simulink model "ifoc_floueOBS"  (R2013a)
settings: Solver=ode45  StartTime=0.0  StopTime=tf  RelTol=1e-3
values from neighbouring files (symbols this model uses):
  A1 = A-(L*C)    [script_param.m]
  B = [(-P*0.85)/J;0]    [script_param.m]
  Cr = 0    [script_param.m]
  fr = 0.001    [script_param.m]
  FS = 50    [script_param.m]
  J = 0.2    [script_param.m]
  Lr = 0.1568    [script_param.m]
  Ls = 0.1568    [script_param.m]
  M = 0.15    [script_param.m]
  mm = L    [script_param.m]
  P = 2    [script_param.m]
  Rr = 1.8    [script_param.m]
  Rs = 1.2    [script_param.m]
  tcr = 3    [script_param.m]
  US = 230    [script_param.m]
libraries: fuzblock x3, simulink x1
settings Model: Creator=admin  LastModifiedBy=cyber
settings SolverCC: ZeroCrossControl=DisableAll
settings DebuggingCC: FrameProcessingCompatibilityMsg=error
settings GRTTargetCC: CodeReplacementLibrary=C89/C90 (ANSI)

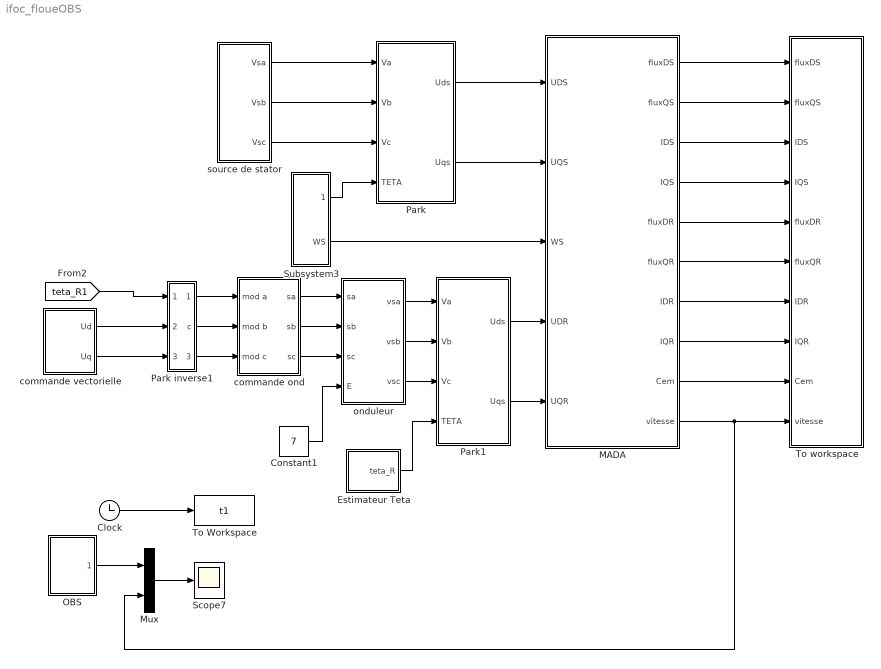
== system ifoc_floueOBS ==
  Clock : Clock
  Constant1 : Constant  Value=7
  Estimateur Teta : Subsystem
  MADA : Subsystem  mask{Rr=Rr, Lr=Lr, Rs=Rs, Ls=Ls, M=M, fr=fr, J=J, P=P, Cr=Cr, t1=tcr}
      mask prompts: t1 "tcr"
  Mux : Mux  Inputs=2
  OBS : Subsystem
  Park : Subsystem
  Park inverse1 : Subsystem
  Park1 : Subsystem
  Scope7 : Scope
      settings: TimeRange=0.0007659594403648384  MaxDataPoints=5000  SaveToWorkspace=off  YMin=153.447  YMax=153.448  SampleTime=-1
  Subsystem3 : Subsystem
  To Workspace : ToWorkspace  VariableName=t1  SaveFormat=Structure  SampleTime=-1
  To workspace : Subsystem
  commande ond : Subsystem
  commande vectorielle : Subsystem
  onduleur : Subsystem
  source de stator : Subsystem
  wires:
  Clock/1 -> To Workspace/1
  commande ond/1(sa) -> onduleur/1(sa)
  commande ond/2(sb) -> onduleur/2(sb)
  commande ond/3(sc) -> onduleur/3(sc)
  Constant1/1 -> onduleur/4(E)
  Park/1(Uds) -> MADA/1(UDS)
  Park/2(Uqs) -> MADA/2(UQS)
  source de stator/1(Vsa) -> Park/1("Va ")
  source de stator/2(Vsb) -> Park/2(Vb)
  source de stator/3(Vsc) -> Park/3(Vc)
  onduleur/1(vsa) -> Park1/1("Va ")
  onduleur/2(vsb) -> Park1/2(Vb)
  onduleur/3(vsc) -> Park1/3(Vc)
  Subsystem3/1(teta_S) -> Park/4(TETA)
  Estimateur Teta/1(teta_R) -> Park1/4(TETA)
  Subsystem3/2(WS) -> MADA/3(WS)
  Park1/1(Uds) -> MADA/4(UDR)
  Park1/2(Uqs) -> MADA/5(UQR)
  Park inverse1/1(a) -> commande ond/1(mod a)
  Park inverse1/2(c) -> commande ond/2(mod b)
  Park inverse1/3(b) -> commande ond/3(mod c)
  commande vectorielle/1(Ud) -> Park inverse1/2(d)
  commande vectorielle/2(Uq) -> Park inverse1/3(q)
  [teta_R1] -> Park inverse1/1(Teta)
  MADA/9(Cem) -> To workspace/9(Cem)
  MADA/8(IQR) -> To workspace/8(IQR)
  MADA/7(IDR) -> To workspace/7(IDR)
  MADA/6(fluxQR) -> To workspace/6(fluxQR)
  MADA/5(fluxDR) -> To workspace/5(fluxDR)
  MADA/4(IQS) -> To workspace/4(IQS)
  MADA/3(IDS) -> To workspace/3(IDS)
  MADA/2(fluxQS) -> To workspace/2(fluxQS)
  MADA/1(fluxDS) -> To workspace/1(fluxDS)
  MADA/10(vitesse) -> Mux/2, To workspace/10(vitesse)
  OBS/1(vit OBS) -> Mux/1
  Mux/1 -> Scope7/1

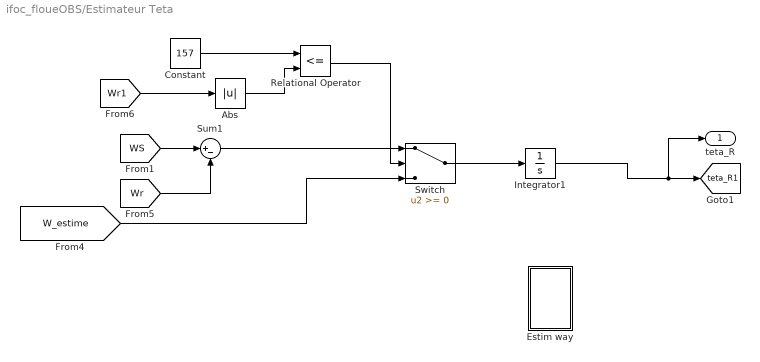
== system ifoc_floueOBS/Estimateur Teta ==
  Abs : Abs
  Constant : Constant  Value=157
  Estim way : Subsystem
  Integrator1 : Integrator
  Relational Operator : RelationalOperator  Operator=<=  OutDataTypeStr=boolean
  Sum1 : Sum  Inputs=|+-
  Switch : Switch
  teta_R : Outport
  tag scope: teta_R1=global
  wires:
  Integrator1/1 -> teta_R/1, [teta_R1]
  [WS] -> Sum1/1
  Constant/1 -> Relational Operator/1
  Relational Operator/1 -> Switch/2
  [W_estime] -> Switch/3
  [Wr1] -> Abs/1
  [Wr] -> Sum1/2
  Sum1/1 -> Switch/1
  Abs/1 -> Relational Operator/2
  Switch/1 -> Integrator1/1

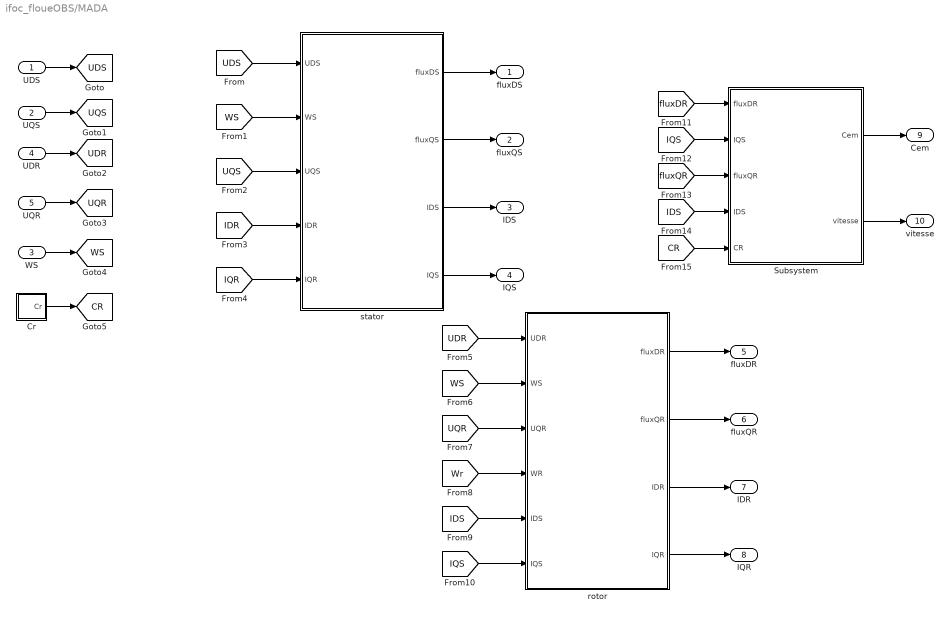
== system ifoc_floueOBS/MADA ==
  UDS : Inport
  UQS : Inport  Port=2
  WS : Inport  Port=3
  UDR : Inport  Port=4
  UQR : Inport  Port=5
  Cr : Subsystem
  Subsystem : Subsystem
  rotor : Subsystem
  stator : Subsystem
  fluxDS : Outport
  fluxQS : Outport  Port=2
  IDS : Outport  Port=3
  IQS : Outport  Port=4
  fluxDR : Outport  Port=5
  fluxQR : Outport  Port=6
  IDR : Outport  Port=7
  IQR : Outport  Port=8
  Cem : Outport  Port=9
  vitesse : Outport  Port=10
  tag scope: CR=global, UDR=global, UDS=global, UQR=global, UQS=global, WS=global
  wires:
  UDS/1 -> [UDS]
  UQS/1 -> [UQS]
  UDR/1 -> [UDR]
  WS/1 -> [WS]
  stator/1(fluxDS) -> fluxDS/1
  stator/2(fluxQS) -> fluxQS/1
  stator/3(IDS) -> IDS/1
  stator/4(IQS) -> IQS/1
  Subsystem/1(Cem) -> Cem/1
  Subsystem/2(vitesse) -> vitesse/1
  rotor/1(fluxDR) -> fluxDR/1
  rotor/2(fluxQR) -> fluxQR/1
  rotor/3(IDR) -> IDR/1
  rotor/4(IQR) -> IQR/1
  [UDS] -> stator/1(UDS)
  [WS] -> stator/2(WS)
  [UQS] -> stator/3(UQS)
  [IDR] -> stator/4(IDR)
  [IQR] -> stator/5(IQR)
  [UDR] -> rotor/1(UDR)
  [WS] -> rotor/2(WS)
  [UQR] -> rotor/3(UQR)
  [Wr] -> rotor/4(WR)
  [IDS] -> rotor/5(IDS)
  [IQS] -> rotor/6(IQS)
  [fluxDR] -> Subsystem/1(fluxDR)
  [IQS] -> Subsystem/2(IQS)
  [fluxQR] -> Subsystem/3(fluxQR)
  [IDS] -> Subsystem/4(IDS)
  [CR] -> Subsystem/5(CR)
  Cr/1(Cr) -> [CR]
  UQR/1 -> [UQR]

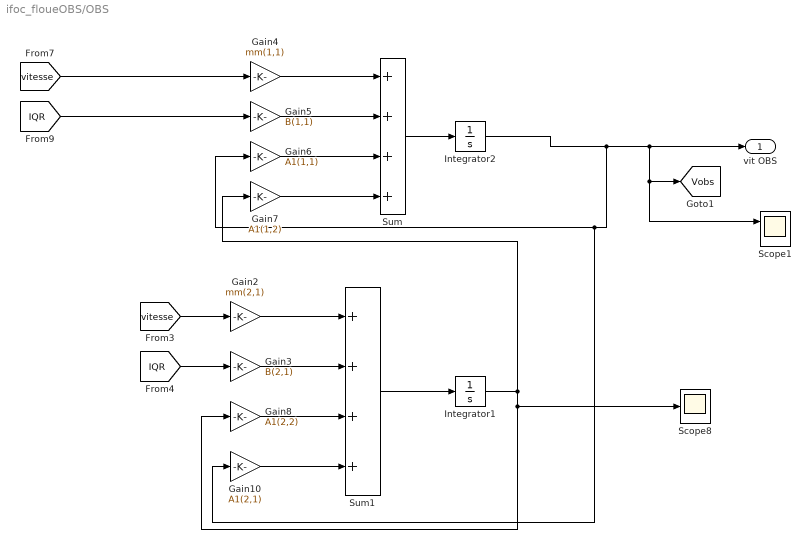
== system ifoc_floueOBS/OBS ==
  Gain10 : Gain  Gain=A1(2,1)
  Gain2 : Gain  Gain=mm(2,1)
  Gain3 : Gain  Gain=B(2,1)
  Gain4 : Gain  Gain=mm(1,1)
  Gain5 : Gain  Gain=B(1,1)
  Gain6 : Gain  Gain=A1(1,1)
  Gain7 : Gain  Gain=A1(1,2)
  Gain8 : Gain  Gain=A1(2,2)
  Integrator1 : Integrator
  Integrator2 : Integrator
  Scope1 : Scope  NumInputPorts=2
      settings: TimeRange=0.0007659594403648384  MaxDataPoints=5000  SaveToWorkspace=off  SaveName=ScopeData31  YMin=153.447~-5  YMax=153.448~5  SampleTime=-1
  Scope8 : Scope
      settings: TimeRange=0.0007659594403648384  MaxDataPoints=5000  SaveToWorkspace=off  SaveName=ScopeData43  YMin=156.9  YMax=157  SampleTime=-1
  Sum : Sum  Inputs=++++
  Sum1 : Sum  Inputs=++++
  vit OBS : Outport
  tag scope: Vobs=global
  wires:
  [vitesse] -> Gain4/1
  [IQR] -> Gain5/1
  Sum/1 -> Integrator2/1
  Integrator2/1 -> Gain10/1, Gain6/1, Scope1/1, [Vobs], vit OBS/1
  Gain7/1 -> Sum/4
  Gain6/1 -> Sum/3
  Gain5/1 -> Sum/2
  Gain4/1 -> Sum/1
  Sum1/1 -> Integrator1/1
  Integrator1/1 -> Gain7/1, Gain8/1, Scope8/1
  [IQR] -> Gain3/1
  Gain3/1 -> Sum1/2
  Gain8/1 -> Sum1/3
  Gain10/1 -> Sum1/4
  [vitesse] -> Gain2/1
  Gain2/1 -> Sum1/1

== system ifoc_floueOBS/Park ==
  "Va " : Inport
  Vb : Inport  Port=2
  Vc : Inport  Port=3
  TETA : Inport  Port=4
  Scope : Scope  NumInputPorts=2
      settings: TimeRange=0.02  LimitDataPoints=on  MaxDataPoints=5000  SaveToWorkspace=off  SaveName=ScopeData  YMin=-0.1~-9.311418685121105e+25  YMax=1~-7.437818033787908e+25  SampleTime=-1
  Transformation de Park : Subsystem
  Uds : Outport
  Uqs : Outport  Port=2
  wires:
  Transformation de Park/2(q) -> Uqs/1, Scope/2
  Transformation de Park/1(d) -> Uds/1, Scope/1
  "Va "/1 -> Transformation de Park/1(Va)
  Vb/1 -> Transformation de Park/2(Vb)
  Vc/1 -> Transformation de Park/3(Vc)
  TETA/1 -> Transformation de Park/4(TETA)

== system ifoc_floueOBS/Park inverse1 ==
  Teta : Inport
  d : Inport  Port=2
  q : Inport  Port=3
  Transformer alpha/betta : Subsystem
  Transformer dq : Subsystem
  a : Outport
  c : Outport  Port=2
  b : Outport  Port=3
  wires:
  q/1 -> Transformer alpha/betta/3(Iq)
  d/1 -> Transformer alpha/betta/2(Id)
  Teta/1 -> Transformer alpha/betta/1(Teta)
  Transformer dq/3(Ic) -> c/1
  Transformer dq/2(Ib) -> b/1
  Transformer dq/1(Ia) -> a/1
  Transformer alpha/betta/2(Xbeta) -> Transformer dq/2(Xbeta)
  Transformer alpha/betta/1(Xalpha) -> Transformer dq/1(Xalpha)

== system ifoc_floueOBS/Park1 ==
  "Va " : Inport
  Vb : Inport  Port=2
  Vc : Inport  Port=3
  TETA : Inport  Port=4
  Scope : Scope  NumInputPorts=2
      settings: TimeRange=0.02  LimitDataPoints=on  MaxDataPoints=5000  SaveToWorkspace=off  SaveName=ScopeData  YMin=-0.1~-9.311418685121105e+25  YMax=1~-7.437818033787908e+25  SampleTime=-1
  Transformation de Park : Subsystem
  Uds : Outport
  Uqs : Outport  Port=2
  wires:
  TETA/1 -> Transformation de Park/4(TETA)
  Vc/1 -> Transformation de Park/3(Vc)
  Vb/1 -> Transformation de Park/2(Vb)
  "Va "/1 -> Transformation de Park/1(Va)
  Transformation de Park/1(d) -> Scope/1, Uds/1
  Transformation de Park/2(q) -> Scope/2, Uqs/1

== system ifoc_floueOBS/Subsystem3 ==
  Constant2 : Constant  Value=2*pi*50
  Integrator2 : Integrator
  teta_S : Outport
  WS : Outport  Port=2
  tag scope: teta_S=global
  wires:
  Integrator2/1 -> [teta_S], teta_S/1
  Constant2/1 -> Integrator2/1
  [Wr1] -> WS/1

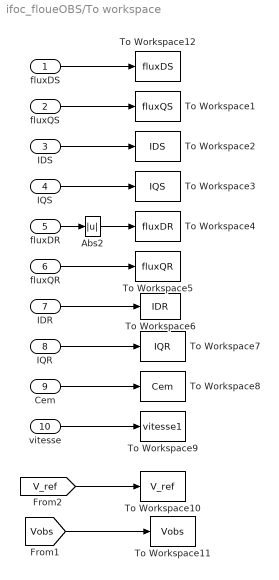
== system ifoc_floueOBS/To workspace ==
  fluxDS : Inport
  fluxQS : Inport  Port=2
  IDS : Inport  Port=3
  IQS : Inport  Port=4
  fluxDR : Inport  Port=5
  fluxQR : Inport  Port=6
  IDR : Inport  Port=7
  IQR : Inport  Port=8
  Cem : Inport  Port=9
  vitesse : Inport  Port=10
  Abs2 : Abs
  To Workspace1 : ToWorkspace  VariableName=fluxQS  SaveFormat=Structure  SampleTime=-1
  To Workspace10 : ToWorkspace  VariableName=V_ref  SaveFormat=Structure  SampleTime=-1
  To Workspace11 : ToWorkspace  VariableName=Vobs  SaveFormat=Structure  SampleTime=-1
  To Workspace12 : ToWorkspace  VariableName=fluxDS  SaveFormat=Structure  SampleTime=-1
  To Workspace2 : ToWorkspace  VariableName=IDS  SaveFormat=Structure  SampleTime=-1
  To Workspace3 : ToWorkspace  VariableName=IQS  SaveFormat=Structure  SampleTime=-1
  To Workspace4 : ToWorkspace  VariableName=fluxDR  SaveFormat=Structure  SampleTime=-1
  To Workspace5 : ToWorkspace  VariableName=fluxQR  SaveFormat=Structure  SampleTime=-1
  To Workspace6 : ToWorkspace  VariableName=IDR  SaveFormat=Structure  SampleTime=-1
  To Workspace7 : ToWorkspace  VariableName=IQR  SaveFormat=Structure  SampleTime=-1
  To Workspace8 : ToWorkspace  VariableName=Cem  SaveFormat=Structure  SampleTime=-1
  To Workspace9 : ToWorkspace  VariableName=vitesse1  SaveFormat=Structure  SampleTime=-1
  wires:
  fluxDS/1 -> To Workspace12/1
  fluxQS/1 -> To Workspace1/1
  IDS/1 -> To Workspace2/1
  IQS/1 -> To Workspace3/1
  fluxQR/1 -> To Workspace5/1
  IQR/1 -> To Workspace7/1
  Cem/1 -> To Workspace8/1
  vitesse/1 -> To Workspace9/1
  fluxDR/1 -> Abs2/1
  Abs2/1 -> To Workspace4/1
  [V_ref] -> To Workspace10/1
  IDR/1 -> To Workspace6/1
  [Vobs] -> To Workspace11/1

== system ifoc_floueOBS/commande ond ==
  mod a : Inport
  mod b : Inport  Port=2
  mod c : Inport  Port=3
  Data Type Conversion : DataTypeConversion  SaturateOnIntegerOverflow=on  RndMeth=Zero
  Data Type Conversion1 : DataTypeConversion  SaturateOnIntegerOverflow=on  RndMeth=Zero
  Data Type Conversion2 : DataTypeConversion  SaturateOnIntegerOverflow=on  RndMeth=Zero
  Relational Operator : RelationalOperator  OutDataTypeStr=boolean
  Relational Operator1 : RelationalOperator  OutDataTypeStr=boolean
  Relational Operator2 : RelationalOperator  OutDataTypeStr=boolean
  Repeating Sequence : simulink/Sources/Repeating Sequence  rep_seq_t="[0 1e-3/4 1e-3/2 3e-3/4  1e-3]"  rep_seq_y="[0 320 0 -320  0]"
  sa : Outport
  sb : Outport  Port=2
  sc : Outport  Port=3
  wires:
  Repeating Sequence/1 -> Relational Operator1/2, Relational Operator/2, Relational Operator2/2
  mod b/1 -> Relational Operator1/1
  mod c/1 -> Relational Operator2/1
  Relational Operator/1 -> Data Type Conversion/1
  Relational Operator1/1 -> Data Type Conversion1/1
  Relational Operator2/1 -> Data Type Conversion2/1
  Data Type Conversion/1 -> sa/1
  Data Type Conversion1/1 -> sb/1
  Data Type Conversion2/1 -> sc/1
  mod a/1 -> Relational Operator/1

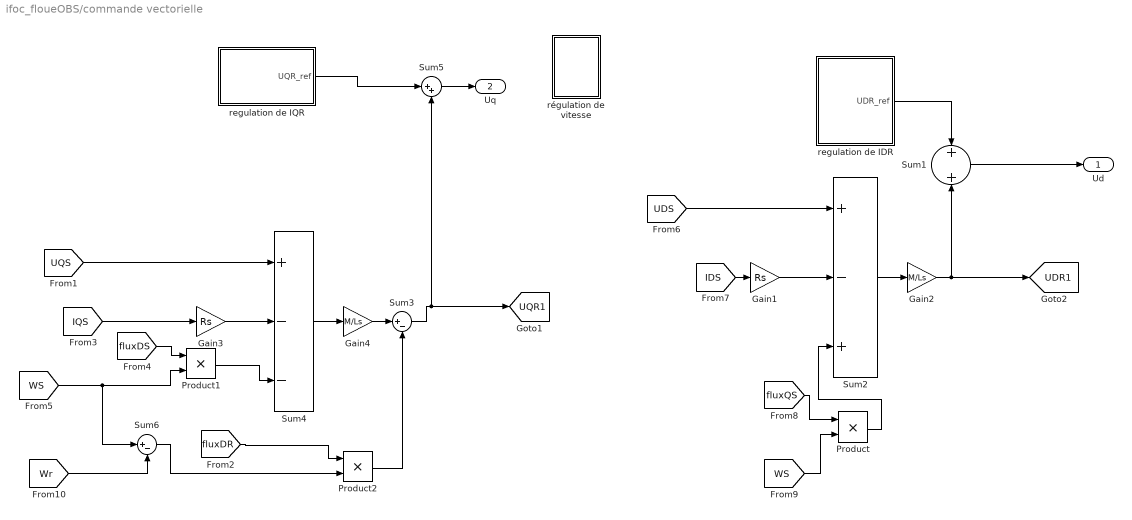
== system ifoc_floueOBS/commande vectorielle ==
  Gain1 : Gain  Gain=Rs
  Gain2 : Gain  Gain=M/Ls
  Gain3 : Gain  Gain=Rs
  Gain4 : Gain  Gain=M/Ls
  Product : Product
  Product1 : Product
  Product2 : Product
  Sum1 : Sum
  Sum2 : Sum  Inputs=+-+
  Sum3 : Sum  Inputs=|+-
  Sum4 : Sum  Inputs=+--
  Sum5 : Sum  Inputs=|++
  Sum6 : Sum  Inputs=|+-
  regulation de IDR : Subsystem
  regulation de IQR : Subsystem
  "régulation de vitesse " : Subsystem
  Ud : Outport
  Uq : Outport  Port=2
  tag scope: UDR1=global, UQR1=global
  wires:
  [fluxQS] -> Product/1
  [IDS] -> Gain1/1
  [UDS] -> Sum2/1
  Gain1/1 -> Sum2/2
  Product/1 -> Sum2/3
  Sum2/1 -> Gain2/1
  [WS] -> Product/2
  Gain2/1 -> Sum1/2, [UDR1]
  Sum1/1 -> Ud/1
  regulation de IDR/1(UDR_ref) -> Sum1/1
  Sum4/1 -> Gain4/1
  Product1/1 -> Sum4/3
  Gain3/1 -> Sum4/2
  [UQS] -> Sum4/1
  [IQS] -> Gain3/1
  [WS] -> Product1/2, Sum6/1
  [fluxDS] -> Product1/1
  Product2/1 -> Sum3/2
  [fluxDR] -> Product2/1
  Gain4/1 -> Sum3/1
  [Wr] -> Sum6/2
  Sum6/1 -> Product2/2
  regulation de IQR/1(UQR_ref) -> Sum5/1
  Sum3/1 -> [UQR1], Sum5/2
  Sum5/1 -> Uq/1

== system ifoc_floueOBS/onduleur ==
  sa : Inport
  sb : Inport  Port=2
  sc : Inport  Port=3
  E : Inport  Port=4
  Mux : Mux
  Va : Fcn  Expr=u(4)*((2/3)*u(1)+(-1/3)*u(2)+(-1/3)*u(3))
  Vb : Fcn  Expr=u(4)*((-1/3)*u(1)+(2/3)*u(2)-(1/3)*u(3))
  Vc : Fcn  Expr=u(4)*((-1/3)*u(1)-(1/3)*u(2)+(2/3)*u(3))
  vsa : Outport
  vsb : Outport  Port=2
  vsc : Outport  Port=3
  wires:
  sa/1 -> Mux/1
  sb/1 -> Mux/2
  sc/1 -> Mux/3
  Mux/1 -> Va/1, Vb/1, Vc/1
  Va/1 -> vsa/1
  Vb/1 -> vsb/1
  Vc/1 -> vsc/1
  E/1 -> Mux/4

== system ifoc_floueOBS/source de stator ==
  Sine Wave : Sin  Amplitude=US  Frequency=FS*2*pi  SampleTime=0
  Sine Wave1 : Sin  Amplitude=US  Frequency=FS*2*pi  Phase=-2*pi/3  SampleTime=0
  Sine Wave2 : Sin  Amplitude=US  Frequency=FS*2*pi  Phase=-4*pi/3  SampleTime=0
  Vsa : Outport
  Vsb : Outport  Port=2
  Vsc : Outport  Port=3
  wires:
  Sine Wave2/1 -> Vsc/1
  Sine Wave1/1 -> Vsb/1
  Sine Wave/1 -> Vsa/1

== system ifoc_floueOBS/Estimateur Teta/Estim way ==
  Constant1 : Constant  Value=0.85
  Gain : Gain  Gain=Rr
  Product : Product  Inputs=*/
  Sum : Sum  Inputs=+-
  tag scope: W_estime=global
  wires:
  [IQR] -> Gain/1
  [UQR] -> Sum/1
  Gain/1 -> Sum/2
  Sum/1 -> Product/1
  Product/1 -> [W_estime]
  Constant1/1 -> Product/2

== system ifoc_floueOBS/MADA/Cr ==
  Step : Step  Time=tcr  After=Cr  SampleTime=0
  Cr : Outport
  wires:
  Step/1 -> Cr/1

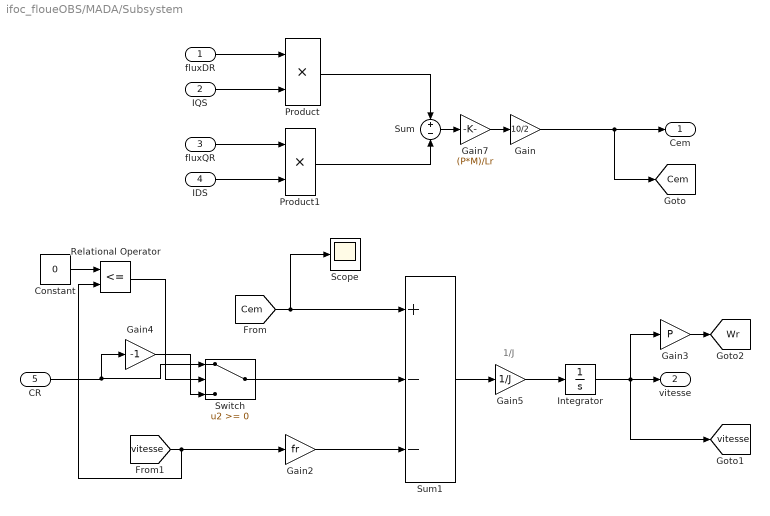
== system ifoc_floueOBS/MADA/Subsystem ==
  note: 1/J
  fluxDR : Inport
  IQS : Inport  Port=2
  fluxQR : Inport  Port=3
  IDS : Inport  Port=4
  CR : Inport  Port=5
  Constant : Constant  Value=0
  Gain : Gain  Gain=10/2
  Gain2 : Gain  Gain=fr
  Gain3 : Gain  Gain=P
  Gain4 : Gain  Gain=-1
  Gain5 : Gain  Gain=1/J
  Gain7 : Gain  Gain=(P*M)/Lr
  Integrator : Integrator
  Product : Product
  Product1 : Product
  Relational Operator : RelationalOperator  Operator=<=  OutDataTypeStr=boolean
  Scope : Scope
      settings: TimeRange=auto  MaxDataPoints=5000  SaveToWorkspace=off  SaveName=ScopeData4  YMin=-10  YMax=10  SampleTime=-1
  Sum : Sum  Inputs=+|-
  Sum1 : Sum  Inputs=+--
  Switch : Switch
  Cem : Outport
  vitesse : Outport  Port=2
  tag scope: Cem=global, Wr=global, vitesse=global
  wires:
  fluxDR/1 -> Product/1
  IQS/1 -> Product/2
  IDS/1 -> Product1/2
  fluxQR/1 -> Product1/1
  Sum/1 -> Gain7/1
  Gain/1 -> [Cem], Cem/1
  [vitesse] -> Relational Operator/2, Gain2/1
  Gain3/1 -> [Wr]
  Integrator/1 -> vitesse/1, Gain3/1, [vitesse]
  Constant/1 -> Relational Operator/1
  Relational Operator/1 -> Switch/2
  Gain4/1 -> Switch/3
  Sum1/1 -> Gain5/1
  Gain5/1 -> Integrator/1
  Gain2/1 -> Sum1/3
  Product1/1 -> Sum/2
  Product/1 -> Sum/1
  Gain7/1 -> Gain/1
  [Cem] -> Sum1/1, Scope/1
  CR/1 -> Switch/1, Gain4/1
  Switch/1 -> Sum1/2

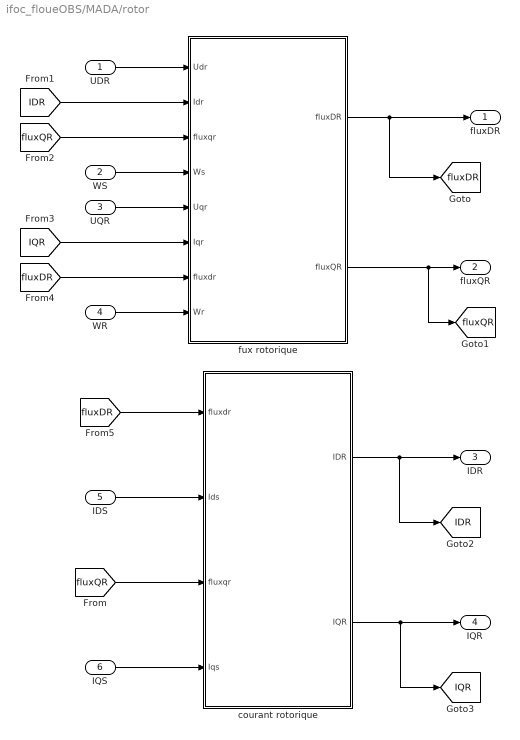
== system ifoc_floueOBS/MADA/rotor ==
  UDR : Inport
  WS : Inport  Port=2
  UQR : Inport  Port=3
  WR : Inport  Port=4
  IDS : Inport  Port=5
  IQS : Inport  Port=6
  courant rotorique : Subsystem
  fux rotorique : Subsystem
  fluxDR : Outport
  fluxQR : Outport  Port=2
  IDR : Outport  Port=3
  IQR : Outport  Port=4
  tag scope: IDR=global, IQR=global, fluxDR=global, fluxQR=global
  wires:
  courant rotorique/1(IDR) -> [IDR], IDR/1
  courant rotorique/2(IQR) -> [IQR], IQR/1
  UDR/1 -> fux rotorique/1(Udr)
  WS/1 -> fux rotorique/4(Ws)
  UQR/1 -> fux rotorique/5(Uqr)
  WR/1 -> fux rotorique/8(Wr)
  IDS/1 -> courant rotorique/2(Ids)
  IQS/1 -> courant rotorique/4(Iqs)
  [IDR] -> fux rotorique/2(Idr)
  [fluxQR] -> fux rotorique/3(fluxqr)
  [IQR] -> fux rotorique/6(Iqr)
  [fluxDR] -> fux rotorique/7(fluxdr)
  [fluxDR] -> courant rotorique/1(fluxdr)
  [fluxQR] -> courant rotorique/3(fluxqr)
  fux rotorique/2(fluxQR) -> [fluxQR], fluxQR/1
  fux rotorique/1(fluxDR) -> fluxDR/1, [fluxDR]

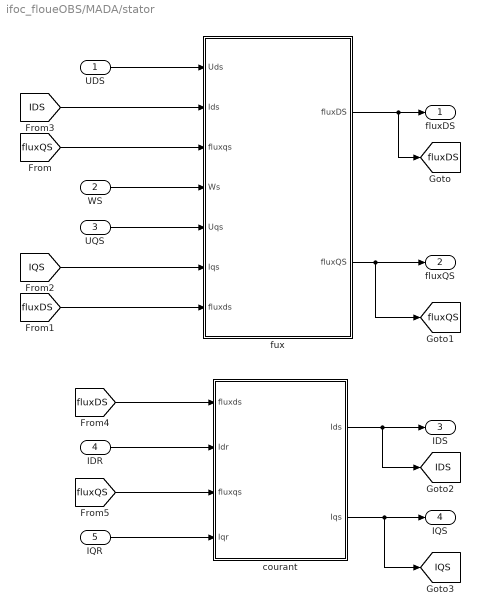
== system ifoc_floueOBS/MADA/stator ==
  UDS : Inport
  WS : Inport  Port=2
  UQS : Inport  Port=3
  IDR : Inport  Port=4
  IQR : Inport  Port=5
  "courant " : Subsystem
  fux : Subsystem
  fluxDS : Outport
  fluxQS : Outport  Port=2
  IDS : Outport  Port=3
  IQS : Outport  Port=4
  tag scope: IDS=global, IQS=global, fluxDS=global, fluxQS=global
  wires:
  fux/1(fluxDS) -> [fluxDS], fluxDS/1
  fux/2(fluxQS) -> [fluxQS], fluxQS/1
  "courant "/1(Ids) -> [IDS], IDS/1
  "courant "/2(Iqs) -> [IQS], IQS/1
  UDS/1 -> fux/1(Uds)
  WS/1 -> fux/4(Ws)
  UQS/1 -> fux/5(Uqs)
  IDR/1 -> "courant "/2(Idr)
  IQR/1 -> "courant "/4(Iqr)
  [fluxQS] -> fux/3(" fluxqs")
  [fluxDS] -> fux/7(" fluxds")
  [IQS] -> fux/6(Iqs)
  [IDS] -> fux/2(Ids)
  [fluxDS] -> "courant "/1(fluxds)
  [fluxQS] -> "courant "/3(fluxqs)

== system ifoc_floueOBS/Park/Transformation de Park ==
  Va : Inport
  Vb : Inport  Port=2
  Vc : Inport  Port=3
  TETA : Inport  Port=4
  Transformer alpha/betta : Subsystem
  Transformer dq : Subsystem
  d : Outport
  q : Outport  Port=2
  wires:
  Va/1 -> Transformer alpha/betta/1(Va)
  Vb/1 -> Transformer alpha/betta/2(Vb)
  Vc/1 -> Transformer alpha/betta/3(Vc)
  Transformer dq/1(d) -> d/1
  Transformer dq/2(q) -> q/1
  Transformer alpha/betta/1(Valpha) -> Transformer dq/1(Valpha)
  Transformer alpha/betta/2(Vbetta) -> Transformer dq/3(Vbetta)
  TETA/1 -> Transformer dq/2(Teta)

== system ifoc_floueOBS/Park inverse1/Transformer alpha//betta ==
  Teta : Inport
  Id : Inport  Port=2
  Iq : Inport  Port=3
  Add : Sum  Inputs=+-
  Product{,1..3} (4 alike) : Product
  Subtract : Sum
  Trigonometric Function : Trigonometry
  Trigonometric Function1 : Trigonometry  Operator=cos
  Xalpha : Outport
  Xbeta : Outport  Port=2
  wires:
  Product3/1 -> Subtract/2
  Product2/1 -> Subtract/1
  Iq/1 -> Product1/2, Product3/1
  Id/1 -> Product2/1, Product/2
  Product1/1 -> Add/2
  Product/1 -> Add/1
  Trigonometric Function/1 -> Product2/2, Product1/1
  Trigonometric Function1/1 -> Product3/2, Product/1
  Teta/1 -> Trigonometric Function/1, Trigonometric Function1/1
  Subtract/1 -> Xbeta/1
  Add/1 -> Xalpha/1

== system ifoc_floueOBS/Park inverse1/Transformer dq ==
  Xalpha : Inport
  Xbeta : Inport  Port=2
  Gain : Gain  Gain=sqrt(2/3)
  Gain1 : Gain  Gain=-1/2
  Gain2 : Gain  Gain=sqrt(3)/2
  Gain3 : Gain  Gain=sqrt(2/3)
  Gain4 : Gain  Gain=sqrt(2/3)
  Subtract : Sum  Inputs=+-
  Subtract1 : Sum
  Ia : Outport
  Ib : Outport  Port=2
  Ic : Outport  Port=3
  wires:
  Gain4/1 -> Ic/1
  Subtract/1 -> Gain4/1
  Gain3/1 -> Ib/1
  Subtract1/1 -> Gain3/1
  Gain2/1 -> Subtract/2, Subtract1/2
  Xbeta/1 -> Gain2/1
  Gain1/1 -> Subtract1/1, Subtract/1
  Xalpha/1 -> Gain1/1, Gain/1
  Gain/1 -> Ia/1

== system ifoc_floueOBS/Park1/Transformation de Park ==
  Va : Inport
  Vb : Inport  Port=2
  Vc : Inport  Port=3
  TETA : Inport  Port=4
  Transformer alpha/betta : Subsystem
  Transformer dq : Subsystem
  d : Outport
  q : Outport  Port=2
  wires:
  TETA/1 -> Transformer dq/2(Teta)
  Transformer dq/2(q) -> q/1
  Transformer dq/1(d) -> d/1
  Vc/1 -> Transformer alpha/betta/3(Vc)
  Vb/1 -> Transformer alpha/betta/2(Vb)
  Va/1 -> Transformer alpha/betta/1(Va)
  Transformer alpha/betta/1(Valpha) -> Transformer dq/1(Valpha)
  Transformer alpha/betta/2(Vbetta) -> Transformer dq/3(Vbetta)

== system ifoc_floueOBS/commande vectorielle/regulation de IDR ==
  Constant : Constant  Value=0
  Derivative : Derivative
  Fuzzy Logic Controller : fuzblock/Fuzzy Logic  Controller  fis=fuzzy5fnc
  Gain : Gain  Gain=0.25
  Gain1 : Gain  Gain=0.5
  Gain2 : Gain  Gain=0.1
  Integrator : Integrator
  Mux : Mux  Inputs=2
  Sum : Sum  Inputs=|+-
  UDR_ref : Outport
  tag scope: UDR_ref=global
  wires:
  Constant/1 -> Sum/1
  [IDR] -> Sum/2
  Mux/1 -> Fuzzy Logic Controller/1
  Sum/1 -> Derivative/1, Gain1/1
  Integrator/1 -> [UDR_ref], UDR_ref/1
  Fuzzy Logic Controller/1 -> Gain/1
  Gain/1 -> Integrator/1
  Gain1/1 -> Mux/1
  Derivative/1 -> Gain2/1
  Gain2/1 -> Mux/2

== system ifoc_floueOBS/commande vectorielle/regulation de IQR ==
  Derivative : Derivative
  Fuzzy Logic Controller : fuzblock/Fuzzy Logic  Controller  fis=fuzzy5fnc
  Gain : Gain  Gain=0.25
  Gain1 : Gain  Gain=0.1
  Gain2 : Gain  Gain=0.5
  Integrator : Integrator
  Mux : Mux  Inputs=2
  Sum : Sum  Inputs=|+-
  UQR_ref : Outport
  tag scope: UQR_ref=global
  wires:
  [IqR_ref] -> Sum/1
  [IQR] -> Sum/2
  Integrator/1 -> [UQR_ref], UQR_ref/1
  Mux/1 -> Fuzzy Logic Controller/1
  Sum/1 -> Gain2/1, Derivative/1
  Gain2/1 -> Mux/1
  Derivative/1 -> Gain1/1
  Gain1/1 -> Mux/2
  Fuzzy Logic Controller/1 -> Gain/1
  Gain/1 -> Integrator/1

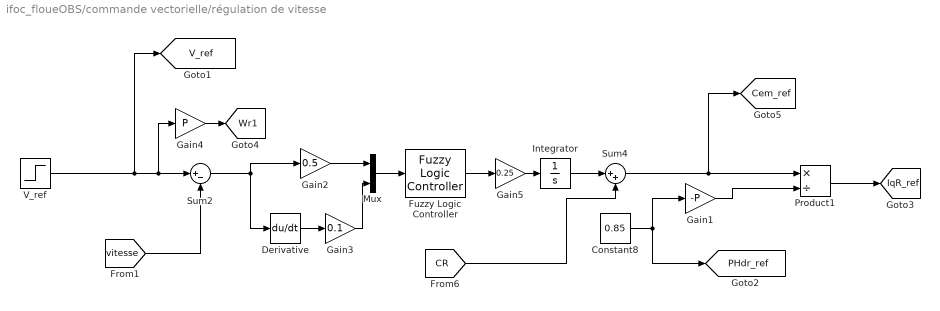
== system ifoc_floueOBS/commande vectorielle/régulation de vitesse  ==
  Constant8 : Constant  Value=0.85
  Derivative : Derivative
  Fuzzy Logic Controller : fuzblock/Fuzzy Logic  Controller  fis=memo22
  Gain1 : Gain  Gain=-P
  Gain2 : Gain  Gain=0.5
  Gain3 : Gain  Gain=0.1
  Gain4 : Gain  Gain=P
  Gain5 : Gain  Gain=0.25
  Integrator : Integrator
  Mux : Mux  Inputs=2
  Product1 : Product  Inputs=*/
  Sum2 : Sum  Inputs=|+-
  Sum4 : Sum  Inputs=|++
  V_ref : Step  Time=2  Before=156  After=156  SampleTime=0
  tag scope: Cem_ref=global, IqR_ref=global, PHdr_ref=global, V_ref=global, Wr1=global
  wires:
  Gain4/1 -> [Wr1]
  [vitesse] -> Sum2/2
  Sum4/1 -> [Cem_ref], Product1/1
  [CR] -> Sum4/2
  Constant8/1 -> Gain1/1, [PHdr_ref]
  Product1/1 -> [IqR_ref]
  Gain1/1 -> Product1/2
  V_ref/1 -> Sum2/1, Gain4/1, [V_ref]
  Integrator/1 -> Sum4/1
  Sum2/1 -> Derivative/1, Gain2/1
  Mux/1 -> Fuzzy Logic Controller/1
  Gain2/1 -> Mux/1
  Derivative/1 -> Gain3/1
  Gain3/1 -> Mux/2
  Fuzzy Logic Controller/1 -> Gain5/1
  Gain5/1 -> Integrator/1

== system ifoc_floueOBS/MADA/rotor/courant rotorique ==
  fluxdr : Inport
  Ids : Inport  Port=2
  fluxqr : Inport  Port=3
  Iqs : Inport  Port=4
  Gain1 : Gain  Gain=M
  Gain2 : Gain  Gain=1/Lr
  Gain4 : Gain  Gain=M
  Gain5 : Gain  Gain=1/Lr
  Sum : Sum  Inputs=+|-
  Sum1 : Sum  Inputs=+|-
  IDR : Outport
  IQR : Outport  Port=2
  wires:
  fluxdr/1 -> Sum/1
  Gain1/1 -> Sum/2
  Sum/1 -> Gain2/1
  Ids/1 -> Gain1/1
  fluxqr/1 -> Sum1/1
  Sum1/1 -> Gain5/1
  Iqs/1 -> Gain4/1
  Gain5/1 -> IQR/1
  Gain4/1 -> Sum1/2
  Gain2/1 -> IDR/1

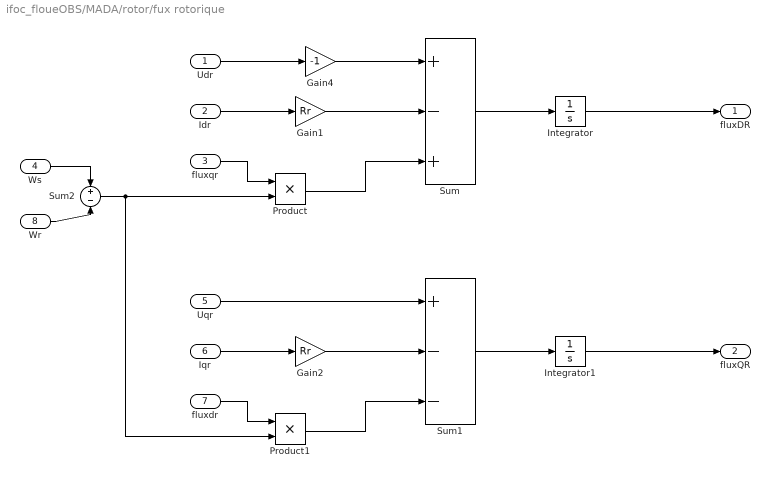
== system ifoc_floueOBS/MADA/rotor/fux rotorique ==
  Udr : Inport
  Idr : Inport  Port=2
  fluxqr : Inport  Port=3
  Ws : Inport  Port=4
  Uqr : Inport  Port=5
  Iqr : Inport  Port=6
  fluxdr : Inport  Port=7
  Wr : Inport  Port=8
  Gain1 : Gain  Gain=Rr
  Gain2 : Gain  Gain=Rr
  Gain4 : Gain  Gain=-1
  Integrator : Integrator
  Integrator1 : Integrator
  Product : Product
  Product1 : Product
  Sum : Sum  Inputs=+-+
  Sum1 : Sum  Inputs=+--
  Sum2 : Sum  Inputs=+|-
  fluxDR : Outport
  fluxQR : Outport  Port=2
  wires:
  Idr/1 -> Gain1/1
  Udr/1 -> Gain4/1
  Gain1/1 -> Sum/2
  fluxqr/1 -> Product/1
  Product/1 -> Sum/3
  Sum/1 -> Integrator/1
  Iqr/1 -> Gain2/1
  Gain2/1 -> Sum1/2
  fluxdr/1 -> Product1/1
  Product1/1 -> Sum1/3
  Sum1/1 -> Integrator1/1
  Integrator1/1 -> fluxQR/1
  Ws/1 -> Sum2/1
  Wr/1 -> Sum2/2
  Sum2/1 -> Product1/2, Product/2
  Uqr/1 -> Sum1/1
  Integrator/1 -> fluxDR/1
  Gain4/1 -> Sum/1

== system ifoc_floueOBS/MADA/stator/courant  ==
  fluxds : Inport
  Idr : Inport  Port=2
  fluxqs : Inport  Port=3
  Iqr : Inport  Port=4
  Gain1 : Gain  Gain=M
  Gain2 : Gain  Gain=1/Ls
  Gain4 : Gain  Gain=M
  Gain5 : Gain  Gain=1/Ls
  Sum : Sum  Inputs=+|-
  Sum1 : Sum  Inputs=+|-
  Ids : Outport
  Iqs : Outport  Port=2
  wires:
  fluxds/1 -> Sum/1
  Gain1/1 -> Sum/2
  Sum/1 -> Gain2/1
  Idr/1 -> Gain1/1
  Gain2/1 -> Ids/1
  fluxqs/1 -> Sum1/1
  Gain4/1 -> Sum1/2
  Sum1/1 -> Gain5/1
  Iqr/1 -> Gain4/1
  Gain5/1 -> Iqs/1

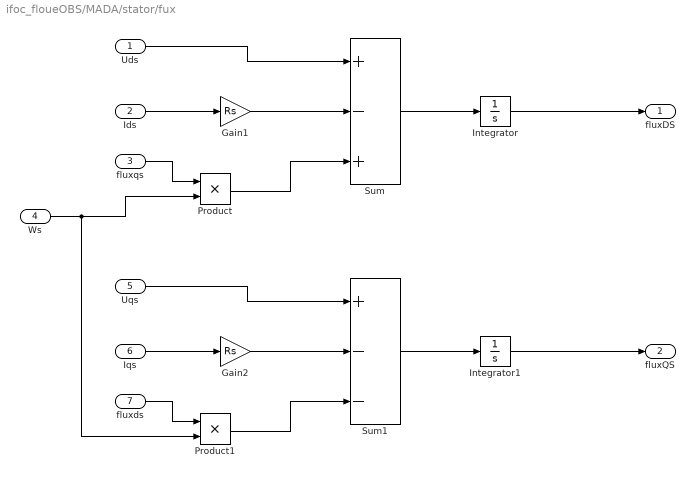
== system ifoc_floueOBS/MADA/stator/fux ==
  Uds : Inport
  Ids : Inport  Port=2
  " fluxqs" : Inport  Port=3
  Ws : Inport  Port=4
  Uqs : Inport  Port=5
  Iqs : Inport  Port=6
  " fluxds" : Inport  Port=7
  Gain1 : Gain  Gain=Rs
  Gain2 : Gain  Gain=Rs
  Integrator : Integrator  ZeroCross=off
  Integrator1 : Integrator
  Product : Product
  Product1 : Product
  Sum : Sum  Inputs=+-+
  Sum1 : Sum  Inputs=+--
  fluxDS : Outport
  fluxQS : Outport  Port=2
  wires:
  Ids/1 -> Gain1/1
  " fluxqs"/1 -> Product/1
  Sum/1 -> Integrator/1
  Integrator/1 -> fluxDS/1
  Iqs/1 -> Gain2/1
  " fluxds"/1 -> Product1/1
  Sum1/1 -> Integrator1/1
  Integrator1/1 -> fluxQS/1
  Ws/1 -> Product1/2, Product/2
  Gain1/1 -> Sum/2
  Gain2/1 -> Sum1/2
  Product/1 -> Sum/3
  Product1/1 -> Sum1/3
  Uds/1 -> Sum/1
  Uqs/1 -> Sum1/1

== system ifoc_floueOBS/Park/Transformation de Park/Transformer alpha//betta ==
  Va : Inport
  Vb : Inport  Port=2
  Vc : Inport  Port=3
  Add : Sum  Inputs=+++
  Gain : Gain  Gain=-1/2
  Gain1 : Gain  Gain=-1/2
  Gain2 : Gain  Gain=sqrt(2/3)
  Gain3 : Gain  Gain=sqrt(2/3)
  Gain4 : Gain  Gain=sqrt(3)/2
  Gain5 : Gain  Gain=sqrt(3)/2
  Subtract : Sum  Inputs=+-
  Valpha : Outport
  Vbetta : Outport  Port=2
  wires:
  Va/1 -> Add/1
  Vb/1 -> Gain/1, Gain4/1
  Gain/1 -> Add/2
  Vc/1 -> Gain1/1, Gain5/1
  Gain1/1 -> Add/3
  Add/1 -> Gain2/1
  Gain2/1 -> Valpha/1
  Subtract/1 -> Gain3/1
  Gain3/1 -> Vbetta/1
  Gain4/1 -> Subtract/1
  Gain5/1 -> Subtract/2

== system ifoc_floueOBS/Park/Transformation de Park/Transformer dq ==
  Valpha : Inport
  Teta : Inport  Port=2
  Vbetta : Inport  Port=3
  Add : Sum
  Product{,1..3} (4 alike) : Product
  Subtract : Sum  Inputs=-+
  Trigonometric Function : Trigonometry
  Trigonometric Function1 : Trigonometry  Operator=cos
  d : Outport
  q : Outport  Port=2
  wires:
  Valpha/1 -> Product2/2, Product/1
  Product/1 -> Add/1
  Teta/1 -> Trigonometric Function/1, Trigonometric Function1/1
  Trigonometric Function1/1 -> Product3/1, Product/2
  Trigonometric Function/1 -> Product2/1, Product1/1
  Product1/1 -> Add/2
  Add/1 -> d/1
  Vbetta/1 -> Product3/2, Product1/2
  Product2/1 -> Subtract/1
  Product3/1 -> Subtract/2
  Subtract/1 -> q/1

== system ifoc_floueOBS/Park1/Transformation de Park/Transformer alpha//betta ==
  Va : Inport
  Vb : Inport  Port=2
  Vc : Inport  Port=3
  Add : Sum  Inputs=+++
  Gain : Gain  Gain=-1/2
  Gain1 : Gain  Gain=-1/2
  Gain2 : Gain  Gain=sqrt(2/3)
  Gain3 : Gain  Gain=sqrt(2/3)
  Gain4 : Gain  Gain=sqrt(3)/2
  Gain5 : Gain  Gain=sqrt(3)/2
  Subtract : Sum  Inputs=+-
  Valpha : Outport
  Vbetta : Outport  Port=2
  wires:
  Gain5/1 -> Subtract/2
  Gain4/1 -> Subtract/1
  Gain3/1 -> Vbetta/1
  Subtract/1 -> Gain3/1
  Gain2/1 -> Valpha/1
  Add/1 -> Gain2/1
  Gain1/1 -> Add/3
  Vc/1 -> Gain5/1, Gain1/1
  Gain/1 -> Add/2
  Vb/1 -> Gain4/1, Gain/1
  Va/1 -> Add/1

== system ifoc_floueOBS/Park1/Transformation de Park/Transformer dq ==
  Valpha : Inport
  Teta : Inport  Port=2
  Vbetta : Inport  Port=3
  Add : Sum
  Product{,1..3} (4 alike) : Product
  Subtract : Sum  Inputs=-+
  Trigonometric Function : Trigonometry
  Trigonometric Function1 : Trigonometry  Operator=cos
  d : Outport
  q : Outport  Port=2
  wires:
  Subtract/1 -> q/1
  Product3/1 -> Subtract/2
  Product2/1 -> Subtract/1
  Vbetta/1 -> Product1/2, Product3/2
  Add/1 -> d/1
  Product1/1 -> Add/2
  Trigonometric Function/1 -> Product1/1, Product2/1
  Trigonometric Function1/1 -> Product/2, Product3/1
  Teta/1 -> Trigonometric Function1/1, Trigonometric Function/1
  Product/1 -> Add/1
  Valpha/1 -> Product/1, Product2/2
